simulink model "h2f_175_S2_sil_plant_model"  (R2023a)
settings: Solver=FixedStepAuto  StartTime=0.0  StopTime=10.0  FixedStep=0.02  RelTol=1e-3
PreLoadFcn:
  | addpath(fullfile('h175_model','thermal'))
  | run('thermal_variants_config.m')
undefined symbols (not defined in the file): b_AnodeSens, b_ARP1_SENS, b_ARP2_SENS, b_auxTCP_SENS, b_CathodeSens, b_CBV_SENS, b_CHUBVd_SENS, b_CHUBVw_SENS, b_CSIV_SENS, b_CSOV_SENS, b_EAC_SENS, b_EATBV_SENS, b_ECoolingSens, b_ElectricalSens, b_ETCP_SENS, b_ETV_SENS, b_ISens_BoP, b_mdotSens_EACi, b_pSens_APRVi, b_pSens_ASti, b_pSens_CLSti, b_pSens_ECL, b_RSens_ISOMON, b_Sens_IVT, b_StackRelay_SENS, b_TCP_SENS, b_TCV_SENS, b_ThermalSens, b_TSens_ASVi, b_TSens_CLSti, b_TSens_CLSto, b_TSens_CSti, b_TSens_TCVi, b_USens_StCV, clean_data_AnodeSens, clean_data_auxTCP_SENS, clean_data_CathodeSens, clean_data_EAC_SENS, clean_data_ECoolingSens, clean_data_ElectricalSens, clean_data_pSens_CLSti, clean_data_Sensors, clean_data_TCP_SENS, clean_data_TCV_SENS, clean_data_ThermalSens, clean_data_ThermalSim, clean_data_TSens_CLSti, clean_data_TSens_CLSto, clean_data_TSens_CSti, clean_data_TSens_TCVi, gaussian, init_Parameters, RELAY_STATE, s_I_A_BOP_Get, s_I_A_StN_Get, s_omega_rpm_ARP1_Get, s_omega_rpm_ARP2_Get, s_omega_rpm_EAC_Get, s_p_bara_APRVi_Get, s_p_bara_ASti_Get ... (+64)
libraries: simulink x17, nesl_utility x1
(part 1 of 2)
settings Model: Creator=stefan.notter  LastModifiedBy=stefan.notter
settings OptimizationCC: DefaultUnderspecifiedDataType=single  ReuseModelBlockBuffer=off
settings DebuggingCC: UnitsInconsistencyMsg=none

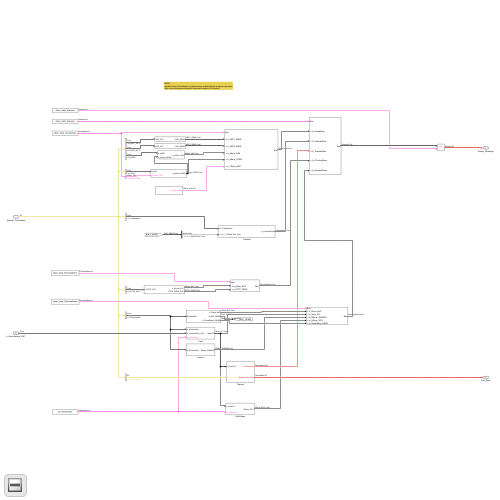
[thumbnail: Simulink's stored preview of the top-level diagram]
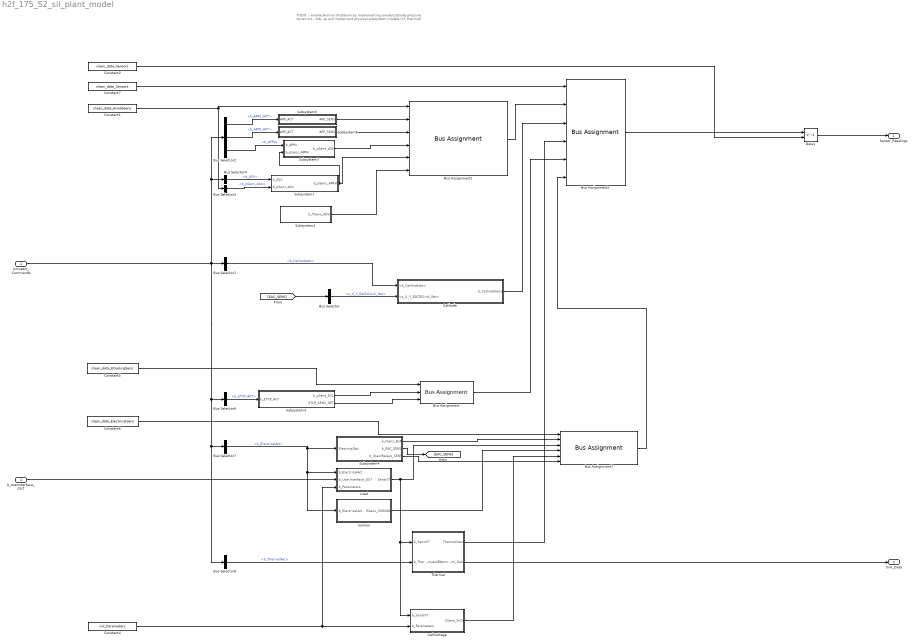
== system h2f_175_S2_sil_plant_model ==
  note: TODO:
      | - enable Normal Shutdown by implementing anode/cathode pressure dynamics
      | - tidy up and implement physical subsystem models (cf. thermal)
  Actuator_Commands : Inport  OutDataTypeStr=Bus: Actuators
  b_UserInterface_OUT : Inport  Port=2  OutDataTypeStr=Bus: UserInterface_OUT
  Bus Assignment : BusAssignment  AssignedSignals=b_pSens_ECL,b_ETCP_SENS
  Bus Assignment1 : BusAssignment  AssignedSignals=b_ARP1_SENS,b_ARP2_SENS,b_pSens_ASti,b_pSens_APRVi,b_TSens_ASVi
  Bus Assignment2 : BusAssignment  AssignedSignals=b_AnodeSens,b_CathodeSens,b_ThermalSens,b_ECoolingSens,b_ElectricalSens
  Bus Assignment7 : BusAssignment  AssignedSignals=b_ISens_BoP,b_Sens_IVT,b_RSens_ISOMON,b_USens_StCV,b_StackRelay_SENS
  Bus Selector : BusSelector  OutputSignals=s_U_V_EACDCLink_Get
  Bus Selector1 : BusSelector  OutputSignals=b_CathodeAct
  Bus Selector2 : BusSelector  OutputSignals=b_AnodeAct.b_ARP1_ACT,b_AnodeAct.b_ARP2_ACT,b_AnodeAct.b_APRV
  Bus Selector3 : BusSelector  OutputSignals=b_pSens_ASti
  Bus Selector4 : BusSelector  OutputSignals=b_AnodeAct.b_ASV
  Bus Selector6 : BusSelector  OutputSignals=b_ECoolingAct.b_ETCP_ACT
  Bus Selector7 : BusSelector  OutputSignals=b_ElectricalAct
  Bus Selector8 : BusSelector  OutputSignals=b_ThermalAct
  Cathode : Subsystem
  CellVoltage : Subsystem
  Constant1 : Constant  Value=clean_data_AnodeSens  OutDataTypeStr=Bus: AnodeSens
  Constant2 : Constant  Value=clean_data_Sensors  OutDataTypeStr=Bus: Sensors
  Constant4 : Constant  Value=init_Parameters  OutDataTypeStr=Bus: Parameters
  Constant5 : Constant  Value=clean_data_ECoolingSens  OutDataTypeStr=Bus: ECoolingSens
  Constant6 : Constant  Value=clean_data_ElectricalSens  OutDataTypeStr=Bus: ElectricalSens
  Constant7 : Constant  Value=clean_data_Sensors  OutDataTypeStr=Bus: Sensors
  Delay : Delay  DelayLength=1  InitialConditionSource=Input port
      settings: InputPortMap=u0,p4
  Isomon : Subsystem
  Load : Subsystem
  Subsystem1 : Subsystem
  Subsystem2 : Subsystem
  Subsystem3 : Subsystem
  Subsystem4 : Subsystem
  Subsystem5 : Subsystem
  Subsystem6 : Subsystem
  Subsystem7 : Subsystem
  Thermal : Subsystem
  Sensor_Readings : Outport  OutDataTypeStr=Bus: Sensors
  Sim_Data : Outport  Port=2  OutDataTypeStr=Bus: ThermalSim
  wires:
  Bus Selector2/2 -> Subsystem6/1(ARP_ACT)  "<b_ARP2_ACT>"
  Constant4/1 -> Load/3(b_Parameters), CellVoltage/2(b_Parameters)
  CellVoltage/1(USens_StCV) -> Bus Assignment7/5
  Isomon/1(RSens_ISOMON) -> Bus Assignment7/4
  Subsystem4/2(b_EAC_SENS) -> [EAC_SENS]
  Constant6/1 -> Bus Assignment7/1
  Subsystem3/2(ETCP_SENS_GET) -> Bus Assignment/3
  Delay/1 -> Sensor_Readings/1
  b_UserInterface_OUT/1 -> Load/2(b_UserInterface_OUT)
  Bus Selector4/1 -> Subsystem1/1(b_ASV)  "<b_ASV>"
  Constant1/1 -> Bus Selector3/1, Bus Assignment1/1
  Load/1(SensIVT) -> CellVoltage/1(b_SensIVT), Thermal/1(b_SensIVT), Bus Assignment7/3
  Bus Assignment2/1 -> Delay/1
  Subsystem3/1(b_pSens_ECL) -> Bus Assignment/2
  Bus Assignment1/1 -> Bus Assignment2/2
  Bus Assignment/1 -> Bus Assignment2/5
  Thermal/1(ThermalSens) -> Bus Assignment2/4
  Bus Selector2/1 -> Subsystem5/1(ARP_ACT)  "<b_ARP1_ACT>"
  Subsystem6/1(ARP_SENS) -> Bus Assignment1/3
  Constant2/1 -> Delay/2
  Subsystem5/1(ARP_SENS) -> Bus Assignment1/2
  Bus Selector8/1 -> Thermal/2(b_ThermalActuators)  "<b_ThermalAct>"
  Actuator_Commands/1 -> Bus Selector1/1, Bus Selector2/1, Bus Selector4/1, Bus Selector8/1, Bus Selector7/1, Bus Selector6/1
  Constant5/1 -> Bus Assignment/1
  Constant7/1 -> Bus Assignment2/1
  Bus Assignment7/1 -> Bus Assignment2/6
  Bus Selector3/1 -> Subsystem1/2(b_pSens_ASti)  "<b_pSens_ASti>"
  Bus Selector7/1 -> Subsystem4/1(ElectricalAct), Isomon/1(b_ElectricalAct), Load/1(b_ElectricalAct)  "<b_ElectricalAct>"
  Bus Selector6/1 -> Subsystem3/1(b_ETCP_ACT)  "<b_ETCP_ACT>"
  Subsystem1/1(b_pSens_APRVi) -> Subsystem7/2(b_pSens_APRVi), Bus Assignment1/5
  Subsystem4/1(b_ISens_BoP) -> Bus Assignment7/2
  [EAC_SENS] -> Bus Selector/1
  Subsystem4/3(b_StackRelays_SENS) -> Bus Assignment7/6
  Subsystem2/1(b_TSens_ASVi) -> Bus Assignment1/6
  Bus Selector2/3 -> Subsystem7/1(b_APRV)  "<b_APRV>"
  Subsystem7/1(b_pSens_ASti) -> Bus Assignment1/4
  Bus Selector1/1 -> Cathode/1(<b_CathodeAct>)  "<b_CathodeAct>"
  Bus Selector/1 -> Cathode/2(<s_U_V_EACDCLink_Get>)  "<s_U_V_EACDCLink_Get>"
  Cathode/1(b_CathodeSens) -> Bus Assignment2/3
  Thermal/2(Thermal_Sim_Data) -> Sim_Data/1

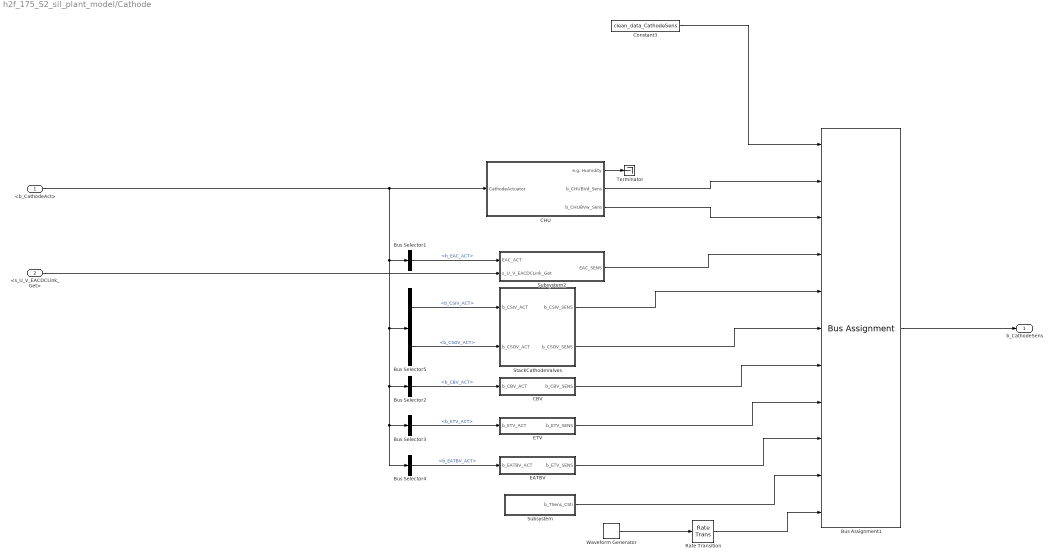
== system h2f_175_S2_sil_plant_model/Cathode ==
  <b_CathodeAct> : Inport
  <s_U_V_EACDCLink_Get> : Inport  Port=2
  Bus Assignment1 : BusAssignment  AssignedSignals=b_CHUBVd_SENS,b_CHUBVw_SENS,b_EAC_SENS,b_CSIV_SENS,b_CSOV_SENS,b_CBV_SENS,b_ETV_SENS,b_EATBV_SENS,b_TSens_CSti,b_mdotSens_EACi.s_mDot_gps_EACi_Get
  Bus Selector1 : BusSelector  OutputSignals=b_EAC_ACT
  Bus Selector2 : BusSelector  OutputSignals=b_CBV_ACT
  Bus Selector3 : BusSelector  OutputSignals=b_ETV_ACT
  Bus Selector4 : BusSelector  OutputSignals=b_EATBV_ACT
  Bus Selector5 : BusSelector  OutputSignals=b_CSIV_ACT,b_CSOV_ACT
  CBV : Subsystem
  CHU : Subsystem
  Constant3 : Constant  Value=clean_data_CathodeSens  OutDataTypeStr=Bus: CathodeSens
  EATBV : Subsystem
  ETV : Subsystem
  Rate Transition : RateTransition
  StackCathodeValves : Subsystem
  Subsystem : Subsystem
  Subsystem2 : Subsystem
  Terminator : Terminator
  Waveform Generator : simulink/Sources/Waveform Generator  OutMin=[]  OutMax=[]  OutDataTypeStr=single  SelectedSignal=1  Signals=gaussian(200,6,23)  BlockNames=MultiportSwitch_9f1233eeb05b44e  SampleTime=0.1
  b_CathodeSens : Outport
  wires:
  Bus Assignment1/1 -> b_CathodeSens/1
  Waveform Generator/1 -> Rate Transition/1
  EATBV/1(b_ETV_SENS) -> Bus Assignment1/9
  Bus Selector4/1 -> EATBV/1(b_EATBV_ACT)  "<b_EATBV_ACT>"
  ETV/1(b_ETV_SENS) -> Bus Assignment1/8
  Subsystem/1(b_TSens_CSti) -> Bus Assignment1/10
  CHU/2(b_CHUBVd_Sens) -> Bus Assignment1/2
  Rate Transition/1 -> Bus Assignment1/11
  StackCathodeValves/1(b_CSIV_SENS) -> Bus Assignment1/5
  StackCathodeValves/2(b_CSOV_SENS) -> Bus Assignment1/6
  Bus Selector2/1 -> CBV/1(b_CBV_ACT)  "<b_CBV_ACT>"
  Bus Selector5/1 -> StackCathodeValves/1(b_CSIV_ACT)  "<b_CSIV_ACT>"
  Bus Selector1/1 -> Subsystem2/1(EAC_ACT)  "<b_EAC_ACT>"
  Bus Selector5/2 -> StackCathodeValves/2(b_CSOV_ACT)  "<b_CSOV_ACT>"
  Bus Selector3/1 -> ETV/1(b_ETV_ACT)  "<b_ETV_ACT>"
  CHU/1(e.g. Humidity) -> Terminator/1
  Subsystem2/1(EAC_SENS) -> Bus Assignment1/4
  <s_U_V_EACDCLink_Get>/1 -> Subsystem2/2(s_U_V_EACDCLink_Get)
  Constant3/1 -> Bus Assignment1/1
  <b_CathodeAct>/1 -> CHU/1(CathodeActuator), Bus Selector1/1, Bus Selector5/1, Bus Selector2/1, Bus Selector3/1, Bus Selector4/1
  CHU/3(b_CHUBVw_Sens) -> Bus Assignment1/3
  CBV/1(b_CBV_SENS) -> Bus Assignment1/7

== system h2f_175_S2_sil_plant_model/CellVoltage ==
  b_SensIVT : Inport  OutDataTypeStr=Bus: Sens_IVT
  b_Parameters : Inport  Port=2  OutDataTypeStr=Bus: Parameters
  Bus Assignment : BusAssignment  AssignedSignals=s_U_V_CVAVG_Get,s_U_V_CVMAX_Get,s_U_V_CVMIN_Get,s_st_enum_StCV_Get
  Bus Selector : BusSelector  OutputSignals=s_U_V_StP_Get
  Bus Selector1 : BusSelector  OutputSignals=b_GEN_Parameters.p_NumberOfCells
  Constant : Constant  Value=struct_USens_StCV  OutDataTypeStr=Bus: USens_StCV
  Divide : Product  Inputs=*/
  Enumerated Constant : simulink/Sources/Enumerated Constant  OutDataTypeStr=Enum: SENS_STATUS  Value=SENS_STATUS.OK  SampleTime=inf
  Gain1 : Gain  Gain=1.01
  Gain2 : Gain  Gain=0.99
  USens_StCV : Outport  OutDataTypeStr=Bus: USens_StCV
  wires:
  Constant/1 -> Bus Assignment/1
  Bus Assignment/1 -> USens_StCV/1
  b_SensIVT/1 -> Bus Selector/1
  Bus Selector/1 -> Divide/1  "<s_U_V_StP_Get>"
  Gain1/1 -> Bus Assignment/3
  Gain2/1 -> Bus Assignment/4
  b_Parameters/1 -> Bus Selector1/1
  Bus Selector1/1 -> Divide/2  "<p_NumberOfCells>"
  Enumerated Constant/1 -> Bus Assignment/5
  Divide/1 -> Gain2/1, Gain1/1, Bus Assignment/2

== system h2f_175_S2_sil_plant_model/Isomon ==
  b_ElectricalAct : Inport  OutDataTypeStr=Bus: ElectricalAct
  Bus Assignment : BusAssignment  AssignedSignals=s_State_enum_ISOMON_Get,s_R_Ohm_ISOMON_Get
  Bus Selector : BusSelector  OutputSignals=b_RSens_ISOMON_ACT.s_State_enum_ISOMON_Set
  Constant : Constant  Value=struct_RSens_ISOMON  OutDataTypeStr=Bus: RSens_ISOMON
  Constant1 : Constant  Value=5e4  OutDataTypeStr=single
  RSens_ISOMON : Outport  OutDataTypeStr=Bus: RSens_ISOMON
  wires:
  Bus Selector/1 -> Bus Assignment/2  "<s_State_enum_ISOMON_Set>"
  b_ElectricalAct/1 -> Bus Selector/1
  Bus Assignment/1 -> RSens_ISOMON/1
  Constant/1 -> Bus Assignment/1
  Constant1/1 -> Bus Assignment/3

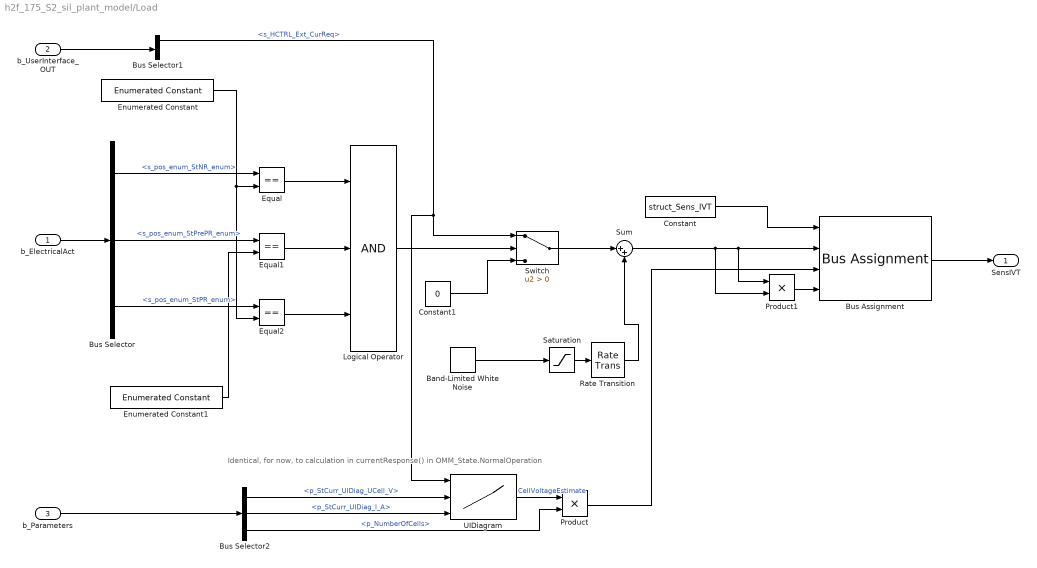
== system h2f_175_S2_sil_plant_model/Load ==
  note: Identical, for now, to calculation in currentResponse() in OMM_State.NormalOperation
  b_ElectricalAct : Inport  OutDataTypeStr=Bus: ElectricalAct
  b_UserInterface_OUT : Inport  Port=2  OutDataTypeStr=Bus: UserInterface_OUT
  b_Parameters : Inport  Port=3  OutDataTypeStr=Bus: Parameters
  Band-Limited White Noise : simulink/Sources/Band-Limited White Noise  Cov=[0.5]  Ts=0.1  seed=[23341]
  Bus Assignment : BusAssignment  AssignedSignals=s_I_A_StN_Get,s_U_V_StP_Get,s_P_W_St_Get
  Bus Selector : BusSelector  OutputSignals=b_StackRelays.s_pos_enum_StNR_enum,b_StackRelays.s_pos_enum_StPrePR_enum,b_StackRelays.s_pos_enum_StPR_enum
  Bus Selector1 : BusSelector  OutputSignals=s_HCTRL_Ext_CurReq,s_HCTRL_Ext_MaxPow
  Bus Selector2 : BusSelector  OutputSignals=b_GEN_Parameters.p_StCurr_UIDiag_UCell_V,b_GEN_Parameters.p_StCurr_UIDiag_I_A,b_GEN_Parameters.p_NumberOfCells
  Constant : Constant  Value=struct_Sens_IVT  OutDataTypeStr=Bus: Sens_IVT
  Constant1 : Constant  Value=0
  Enumerated Constant : simulink/Sources/Enumerated Constant  OutDataTypeStr=Enum: RELAY_STATE  Value=RELAY_STATE.Connected  SampleTime=inf
  Enumerated Constant1 : simulink/Sources/Enumerated Constant  OutDataTypeStr=Enum: RELAY_STATE  Value=RELAY_STATE.Disconnected  SampleTime=inf
  Equal : RelationalOperator  Operator===  OutDataTypeStr=boolean  RndMeth=Simplest  InputSameDT=off
  Equal1 : RelationalOperator  Operator===  OutDataTypeStr=boolean  RndMeth=Simplest  InputSameDT=off
  Equal2 : RelationalOperator  Operator===  OutDataTypeStr=boolean  RndMeth=Simplest  InputSameDT=off
  Logical Operator : Logic  Inputs=3  AllPortsSameDT=off  OutDataTypeStr=boolean
  Product : Product
  Product1 : Product
  Rate Transition : RateTransition
  Saturation : Saturate  UpperLimit=0.4  LowerLimit=-0.4
  Sum : Sum  Inputs=|++  OutDataTypeStr=single
  Switch : Switch  Criteria=u2 > Threshold  SaturateOnIntegerOverflow=off  InputSameDT=off
  UIDiagram : Lookup_n-D  NumberOfTableDimensions=1  BreakpointsForDimension1Source=Input port  BreakpointsForDimension1=[-5:5]  BreakpointsForDimension2Source=Input port  TableSource=Input port  Table=tanh([-5:5])  ExtrapMethod=Clip  UseLastTableValue=on  InternalRulePriority=Speed  RndMeth=Simplest
      settings: InputPortMap=u0,p221,p5
  SensIVT : Outport  OutDataTypeStr=Bus: Sens_IVT
  wires:
  Constant/1 -> Bus Assignment/1
  Bus Assignment/1 -> SensIVT/1
  b_ElectricalAct/1 -> Bus Selector/1
  Constant1/1 -> Switch/3
  Sum/1 -> Product1/2, Product1/1, Bus Assignment/2
  Bus Selector/2 -> Equal1/1  "<s_pos_enum_StPrePR_enum>"
  Bus Selector/3 -> Equal2/1  "<s_pos_enum_StPR_enum>"
  Bus Selector/1 -> Equal/1  "<s_pos_enum_StNR_enum>"
  Equal/1 -> Logical Operator/1
  Equal1/1 -> Logical Operator/2
  Equal2/1 -> Logical Operator/3
  Enumerated Constant/1 -> Equal2/2, Equal/2
  Enumerated Constant1/1 -> Equal1/2
  Logical Operator/1 -> Switch/2
  b_UserInterface_OUT/1 -> Bus Selector1/1
  Bus Selector1/1 -> UIDiagram/1, Switch/1  "<s_HCTRL_Ext_CurReq>"
  b_Parameters/1 -> Bus Selector2/1
  Bus Selector2/2 -> UIDiagram/3  "<p_StCurr_UIDiag_I_A>"
  Bus Selector2/1 -> UIDiagram/2  "<p_StCurr_UIDiag_UCell_V>"
  UIDiagram/1 -> Product/1  "CellVoltageEstimate"
  Bus Selector2/3 -> Product/2  "<p_NumberOfCells>"
  Product/1 -> Bus Assignment/3
  Product1/1 -> Bus Assignment/4
  Band-Limited White Noise/1 -> Saturation/1
  Switch/1 -> Sum/1
  Rate Transition/1 -> Sum/2
  Saturation/1 -> Rate Transition/1

== system h2f_175_S2_sil_plant_model/Subsystem1 ==
  b_ASV : Inport  OutDataTypeStr=Bus: ASV  PortDimensions=1
  b_pSens_ASti : Inport  Port=2  OutDataTypeStr=Bus: pSens_ASti  PortDimensions=1
  Bus Assignment : BusAssignment  AssignedSignals=s_p_bara_APRVi_Get,s_st_enum_APRVi_Get
  Bus Selector : BusSelector  OutputSignals=s_pos_enum_ASV_Set
  Bus Selector1 : BusSelector  OutputSignals=s_p_bara_ASti_Get
  Constant : Constant  Value=struct_pSens_APRVi  OutDataTypeStr=Bus: pSens_APRVi
  Enumerated Constant : simulink/Sources/Enumerated Constant  OutDataTypeStr=Enum: SENS_STATUS  Value=SENS_STATUS.OK  SampleTime=inf
  Multiport Switch : MultiPortSwitch  DataPortOrder=Specify indices  DataPortIndices={DVLV_STATE.Open, DVLV_STATE.Closed}  SaturateOnIntegerOverflow=off  InputSameDT=off
  Sum : Sum  Inputs=|++
  bara : Constant  Value=2.79  OutDataTypeStr=single
  dontJudge : Constant  Value=3  OutDataTypeStr=single
  b_pSens_APRVi : Outport  OutDataTypeStr=Bus: pSens_APRVi
  wires:
  Constant/1 -> Bus Assignment/1
  bara/1 -> Multiport Switch/2
  Enumerated Constant/1 -> Bus Assignment/3
  Bus Selector/1 -> Multiport Switch/1  "<s_pos_enum_ASV_Set>"
  Bus Assignment/1 -> b_pSens_APRVi/1
  Multiport Switch/1 -> Bus Assignment/2
  b_pSens_ASti/1 -> Bus Selector1/1
  Sum/1 -> Multiport Switch/3
  b_ASV/1 -> Bus Selector/1
  Bus Selector1/1 -> Sum/1  "<s_p_bara_ASti_Get>"
  dontJudge/1 -> Sum/2

== system h2f_175_S2_sil_plant_model/Subsystem2 ==
  Bus Assignment : BusAssignment  AssignedSignals=s_T_degC_ASVi_Get,s_st_enum_ASVi_Get
  Constant : Constant  Value=30  OutDataTypeStr=single
  Constant1 : Constant  Value=struct_TSens_ASVi  OutDataTypeStr=Bus: TSens_ASVi
  Enumerated Constant : simulink/Sources/Enumerated Constant  OutDataTypeStr=Enum: SENS_STATUS  Value=SENS_STATUS.OK  SampleTime=inf
  b_TSens_ASVi : Outport
  wires:
  Constant/1 -> Bus Assignment/2
  Enumerated Constant/1 -> Bus Assignment/3
  Constant1/1 -> Bus Assignment/1
  Bus Assignment/1 -> b_TSens_ASVi/1

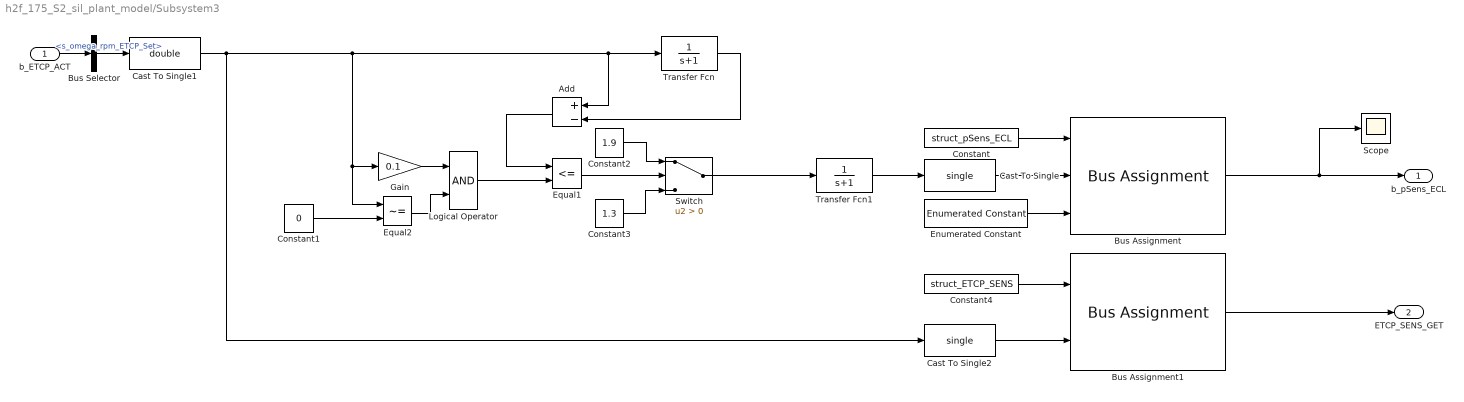
== system h2f_175_S2_sil_plant_model/Subsystem3 ==
  b_ETCP_ACT : Inport  OutDataTypeStr=Bus: ETCP_ACT
  Add : Sum  Inputs=+-
  Bus Assignment : BusAssignment  AssignedSignals=s_p_bara_ECL_Get,s_st_enum_ECL_Get
  Bus Assignment1 : BusAssignment  AssignedSignals=s_omega_rpm_ETCP_Get
  Bus Selector : BusSelector  OutputSignals=s_omega_rpm_ETCP_Set
  Cast To Single : DataTypeConversion  OutDataTypeStr=single  SaturateOnIntegerOverflow=off  RndMeth=Floor
  Cast To Single1 : DataTypeConversion  OutDataTypeStr=double  SaturateOnIntegerOverflow=off  RndMeth=Floor
  Cast To Single2 : DataTypeConversion  OutDataTypeStr=single  SaturateOnIntegerOverflow=off  RndMeth=Floor
  Constant : Constant  Value=struct_pSens_ECL  OutDataTypeStr=Bus: pSens_ECL
  Constant1 : Constant  Value=0
  Constant2 : Constant  Value=1.9
  Constant3 : Constant  Value=1.3
  Constant4 : Constant  Value=struct_ETCP_SENS  OutDataTypeStr=Bus: ETCP_SENS
  Enumerated Constant : simulink/Sources/Enumerated Constant  OutDataTypeStr=Enum: SENS_STATUS  Value=SENS_STATUS.OK  SampleTime=inf
  Equal1 : RelationalOperator  Operator=<=  OutDataTypeStr=boolean  RndMeth=Simplest  InputSameDT=off
  Equal2 : RelationalOperator  Operator=~=  OutDataTypeStr=boolean  RndMeth=Simplest  InputSameDT=off
  Gain : Gain  Gain=0.1
  Logical Operator : Logic  AllPortsSameDT=off  OutDataTypeStr=boolean
  Scope : Scope
  Switch : Switch  Criteria=u2 > Threshold  SaturateOnIntegerOverflow=off  InputSameDT=off
  Transfer Fcn : TransferFcn  Denominator=[1 1]
  Transfer Fcn1 : TransferFcn  Denominator=[1 1]
  b_pSens_ECL : Outport  OutDataTypeStr=Bus: pSens_ECL
  ETCP_SENS_GET : Outport  Port=2  OutDataTypeStr=Bus: ETCP_SENS
  wires:
  Bus Selector/1 -> Cast To Single1/1  "<s_omega_rpm_ETCP_Set>"
  Constant1/1 -> Equal2/2
  Switch/1 -> Transfer Fcn1/1
  b_ETCP_ACT/1 -> Bus Selector/1
  Constant2/1 -> Switch/1
  Logical Operator/1 -> Equal1/2
  Transfer Fcn1/1 -> Cast To Single/1
  Equal2/1 -> Logical Operator/2
  Equal1/1 -> Switch/2
  Constant3/1 -> Switch/3
  Gain/1 -> Logical Operator/1
  Add/1 -> Equal1/1
  Constant4/1 -> Bus Assignment1/1
  Bus Assignment/1 -> Scope/1, b_pSens_ECL/1
  Enumerated Constant/1 -> Bus Assignment/3
  Bus Assignment1/1 -> ETCP_SENS_GET/1
  Constant/1 -> Bus Assignment/1
  Transfer Fcn/1 -> Add/2
  Cast To Single/1 -> Bus Assignment/2
  Cast To Single1/1 -> Cast To Single2/1, Equal2/1, Gain/1, Add/1, Transfer Fcn/1
  Cast To Single2/1 -> Bus Assignment1/2

== system h2f_175_S2_sil_plant_model/Subsystem4 ==
  ElectricalAct : Inport  OutDataTypeStr=Bus: ElectricalAct
  HVRelays : Subsystem
  StackRelays : Subsystem
  b_ISens_BoP : Outport  OutDataTypeStr=Bus: ISens_BoP
  b_EAC_SENS : Outport  Port=2  OutDataTypeStr=Bus: EAC_SENS
  b_StackRelays_SENS : Outport  Port=3  OutDataTypeStr=Bus: StackRelay_SENS
  wires:
  ElectricalAct/1 -> HVRelays/1(ElectricalAct), StackRelays/1(ElectricalAct)
  StackRelays/1(b_ISens_BoP) -> b_ISens_BoP/1
  HVRelays/1(b_EAC_SENS) -> b_EAC_SENS/1
  StackRelays/2(b_StackRelays_SENS) -> b_StackRelays_SENS/1

== system h2f_175_S2_sil_plant_model/Subsystem5 ==
  ARP_ACT : Inport  OutDataTypeStr=Bus: ARP1_ACT  PortDimensions=1
  Bus Assignment : BusAssignment  AssignedSignals=s_omega_rpm_ARP1_Get,s_st_enum_ARP1_Get
  Bus Selector : BusSelector  OutputSignals=s_omega_rpm_ARP1_Set
  Cast To Double : DataTypeConversion  OutDataTypeStr=double  SaturateOnIntegerOverflow=off  RndMeth=Floor
  Cast To Single : DataTypeConversion  OutDataTypeStr=single  SaturateOnIntegerOverflow=off  RndMeth=Floor
  Constant : Constant  Value=struct_ARP1_SENS  OutDataTypeStr=Bus: ARP1_SENS
  Enumerated Constant : simulink/Sources/Enumerated Constant  OutDataTypeStr=Enum: SENS_STATUS  Value=SENS_STATUS.OK  SampleTime=inf
  Transfer Fcn : TransferFcn  Numerator=[4]  Denominator=[1 2 4]
  ARP_SENS : Outport  OutDataTypeStr=Bus: ARP1_SENS  PortDimensions=1
  wires:
  Bus Assignment/1 -> ARP_SENS/1
  Enumerated Constant/1 -> Bus Assignment/3
  Bus Selector/1 -> Cast To Double/1  "<s_omega_rpm_ARP1_Set>"
  ARP_ACT/1 -> Bus Selector/1
  Constant/1 -> Bus Assignment/1
  Transfer Fcn/1 -> Cast To Single/1  "meas"
  Cast To Single/1 -> Bus Assignment/2
  Cast To Double/1 -> Transfer Fcn/1

== system h2f_175_S2_sil_plant_model/Subsystem6 ==
  ARP_ACT : Inport  OutDataTypeStr=Bus: ARP2_ACT  PortDimensions=1
  Bus Assignment : BusAssignment  AssignedSignals=s_omega_rpm_ARP2_Get,s_st_enum_ARP2_Get
  Bus Selector : BusSelector  OutputSignals=s_omega_rpm_ARP2_Set
  Cast To Double : DataTypeConversion  OutDataTypeStr=double  SaturateOnIntegerOverflow=off  RndMeth=Floor
  Cast To Single : DataTypeConversion  OutDataTypeStr=single  SaturateOnIntegerOverflow=off  RndMeth=Floor
  Constant : Constant  Value=struct_ARP2_SENS  OutDataTypeStr=Bus: ARP2_SENS
  Enumerated Constant : simulink/Sources/Enumerated Constant  OutDataTypeStr=Enum: SENS_STATUS  Value=SENS_STATUS.OK  SampleTime=inf
  Transfer Fcn : TransferFcn  Numerator=[4]  Denominator=[1 2 4]
  ARP_SENS : Outport  OutDataTypeStr=Bus: ARP2_SENS  PortDimensions=1
  wires:
  Transfer Fcn/1 -> Cast To Single/1  "meas"
  Enumerated Constant/1 -> Bus Assignment/3
  ARP_ACT/1 -> Bus Selector/1
  Constant/1 -> Bus Assignment/1
  Bus Selector/1 -> Cast To Double/1  "<s_omega_rpm_ARP2_Set>"
  Bus Assignment/1 -> ARP_SENS/1
  Cast To Double/1 -> Transfer Fcn/1
  Cast To Single/1 -> Bus Assignment/2

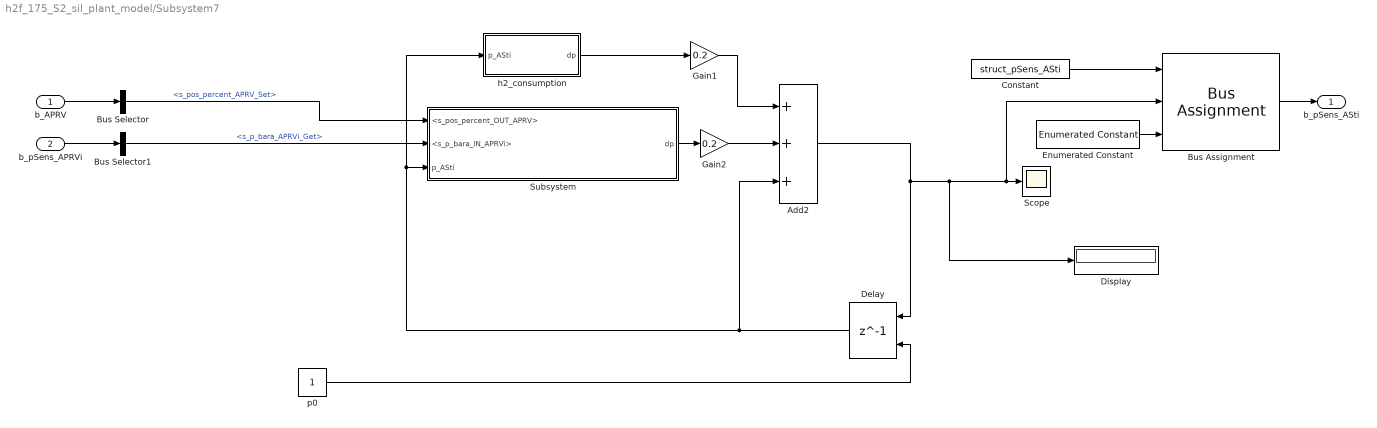
== system h2f_175_S2_sil_plant_model/Subsystem7 ==
  b_APRV : Inport  OutDataTypeStr=Bus: APRV  PortDimensions=1
  b_pSens_APRVi : Inport  Port=2  OutDataTypeStr=Bus: pSens_APRVi  PortDimensions=1
  Add2 : Sum  Inputs=+++
  Bus Assignment : BusAssignment  AssignedSignals=s_p_bara_ASti_Get,s_st_enum_ASti_Get
  Bus Selector : BusSelector  OutputSignals=s_pos_percent_APRV_Set
  Bus Selector1 : BusSelector  OutputSignals=s_p_bara_APRVi_Get
  Constant : Constant  Value=struct_pSens_ASti  OutDataTypeStr=Bus: pSens_ASti
  Delay : Delay  DelayLength=1  InitialConditionSource=Input port
      settings: InputPortMap=u0,p4
  Display : Display
  Enumerated Constant : simulink/Sources/Enumerated Constant  OutDataTypeStr=Enum: SENS_STATUS  Value=SENS_STATUS.OK  SampleTime=inf
  Gain1 : Gain  Gain=0.2
  Gain2 : Gain  Gain=0.2
  Scope : Scope
  Subsystem : Subsystem
  h2_consumption : Subsystem
  p0 : Constant  OutDataTypeStr=single
  b_pSens_ASti : Outport  OutDataTypeStr=Bus: pSens_ASti
  wires:
  Enumerated Constant/1 -> Bus Assignment/3
  h2_consumption/1(dp) -> Gain1/1
  Subsystem/1(dp) -> Gain2/1
  Constant/1 -> Bus Assignment/1
  Bus Selector/1 -> Subsystem/1(<s_pos_percent_OUT_APRV>)  "<s_pos_percent_APRV_Set>"
  Bus Selector1/1 -> Subsystem/2(<s_p_bara_IN_APRVi>)  "<s_p_bara_APRVi_Get>"
  Delay/1 -> h2_consumption/1(p_ASti), Subsystem/3(p_ASti), Add2/3
  p0/1 -> Delay/2
  b_pSens_APRVi/1 -> Bus Selector1/1
  Bus Assignment/1 -> b_pSens_ASti/1
  b_APRV/1 -> Bus Selector/1
  Add2/1 -> Delay/1, Display/1, Scope/1, Bus Assignment/2
  Gain1/1 -> Add2/1
  Gain2/1 -> Add2/2

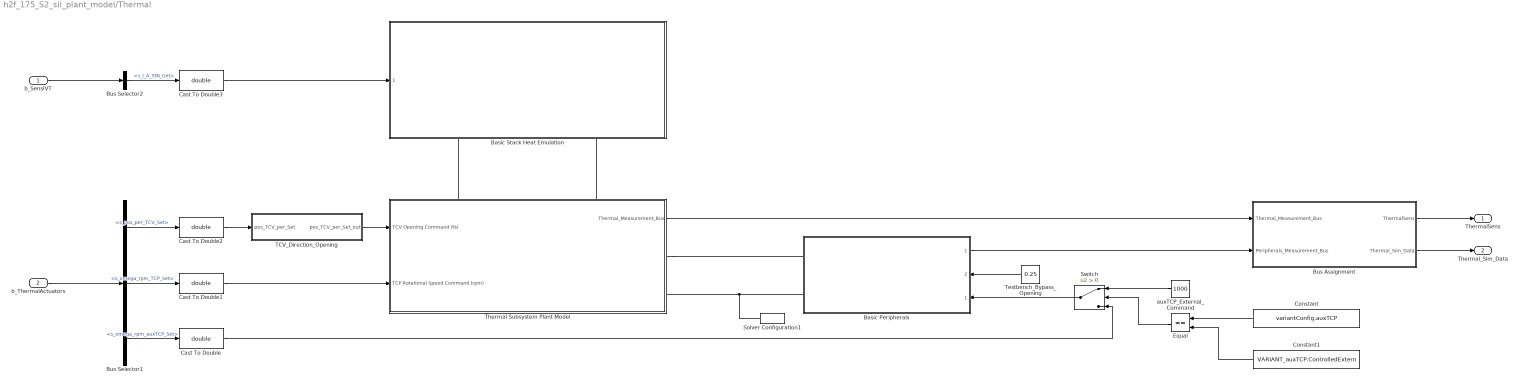
== system h2f_175_S2_sil_plant_model/Thermal ==
  b_SensIVT : Inport
  b_ThermalActuators : Inport  Port=2  OutDataTypeStr=Bus: ThermalAct
  Basic Peripherals : Subsystem  ReferencedSubsystem=thermal_basic_peripherals
      settings: PortSchema="{\"entries\":[{\"content\":{\"sides\":[{\"content\":{\"connectorIds\":[\"LConn1\",\"LConn2\"]},\"type\":\"ConnectorPlacement.EquallySpacedRectSide\",\"uuid\":\"3fb1bffc-06de-43a0-ba54-014616fc6cc1\"},{\"content\":{\"connectorIds\":[\"Out1\",\"In2\",\"In1\"],\"side\":\"RIGHT\"},\"type\":\"ConnectorPlacement.EquallySpacedRectSide\",\"uuid\":\"58405954-0a26-4c47-92cd-2c539f5c2dc2\"},{\"content\":{\"side\":\"TOP\"},\"type\":\"ConnectorPlacement.EquallySpacedRectSide\",\"uuid\":\"fb935e14-bdb8-42f8-ab88-5e819e25323e\"},{\"content\":{\"side\":\"BOTTOM\"},\"type\":\"ConnectorPlacement.EquallySpacedRectSide\",\"uuid\":\"e6e8be2d-a7ad-4d02-9de8-873dcaf650b4\"}]},\"type\":\"ConnectorPlacement.EquallySpacedConnector\",\"uuid\":\"bd863423-caf1-4028-a014-0e522635d1ca\"}],\"packageUris\":[\"http://schema.mathworks.com/mf0/Connector/R2020b\"],\"version\":\"1.0\"}"
  Basic Stack Heat Emulation : Subsystem  ReferencedSubsystem=thermal_stack_heat_emulation
      settings: PortSchema="{\"entries\":[{\"content\":{\"sides\":[{\"content\":{\"connectorIds\":[\"In1\"]},\"type\":\"ConnectorPlacement.EquallySpacedRectSide\",\"uuid\":\"3fb1bffc-06de-43a0-ba54-014616fc6cc1\"},{\"content\":{\"side\":\"RIGHT\"},\"type\":\"ConnectorPlacement.EquallySpacedRectSide\",\"uuid\":\"58405954-0a26-4c47-92cd-2c539f5c2dc2\"},{\"content\":{\"side\":\"TOP\"},\"type\":\"ConnectorPlacement.EquallySpacedRectSide\",\"uuid\":\"fb935e14-bdb8-42f8-ab88-5e819e25323e\"},{\"content\":{\"connectorIds\":[\"RConn1\",\"RConn2\"],\"side\":\"BOTTOM\"},\"type\":\"ConnectorPlacement.EquallySpacedRectSide\",\"uuid\":\"52bc4db1-df79-4132-9e52-2843fbef2d40\"}]},\"type\":\"ConnectorPlacement.EquallySpacedConnector\",\"uuid\":\"bd863423-caf1-4028-a014-0e522635d1ca\"}],\"packageUris\":[\"http://schema.mathworks.com/mf0/Connector/R2020b\"],\"version\":\"1.0\"}"
  Bus Selector1 : BusSelector  OutputSignals=b_TCV_ACT.s_pos_per_TCV_Set,b_TCP_ACT.s_omega_rpm_TCP_Set,b_auxTCP_ACT.s_omega_rpm_auxTCP_Set
  Bus Selector2 : BusSelector  OutputSignals=s_I_A_StN_Get
  Bus Assignment : Subsystem
  Cast To Double{,1..3} (4 alike) : DataTypeConversion  OutDataTypeStr=double  SaturateOnIntegerOverflow=off  RndMeth=Floor
  Constant : Constant  Value=variantConfig.auxTCP
  Constant1 : Constant  Value=VARIANT_auxTCP.ControlledExtern
  Equal : RelationalOperator  Operator===  OutDataTypeStr=boolean  RndMeth=Simplest  InputSameDT=off
  Solver Configuration1 : nesl_utility/Solver Configuration  PhysicalDomain=network_engine_domain  SubClassName=solver  LeftPortType=input  RightPortType=generic  Tones=[]  Harmonics=[]  SimulateNoise=off  Profile=off  UseLocalSampling=off  EnableSwitchedLinearOptims=on  FrequencyDomain=off  UseCCode=off  RelTol=0.001  AbsTol=1e-06  MinStep=1e-09  ToWorkspace=off  RevertToSquareIcSolve=off  NumHomotopyIterations=100  PhasorMode=off  PhasorModeNumHarmonics=1  ConsistencySolver=NEWTON_XTOL_AFTER_FTOL  IndexReductionMethod=DerivativeReplacement  DoDC=off  ResidualTolerance=1e-09  ConsistencyTolSource=GLOBAL  ConsistencyAbsTol=0.001  ConsistencyRelTol=0.001  ConsistencyTolFactor=0.001  UseLocalSolver=on  LocalSolverChoice=NE_BACKWARD_EULER_ADVANCER  ResolveIndetEquations=on  FunctionEvalNumThread=1  LocalSolverSampleTime=0.02  DoFixedCost=on  MaxNonlinIter=3  MaxModeIter=2  ComputeImpulses=off  ImpulseIterations=2  LinearAlgebra=auto  LinearAlgebraNumThread=0  EquationFormulation=NE_TIME_EF  DelaysMemoryBudget=1024  AutomaticFiltering=off  FilteringTimeConstant=0.001  PartitionStorageMethod=AS_NEEDED  PartitionMemoryBudget=1024  PartitionMethod=ROBUST
  Switch : Switch  Criteria=u2 > Threshold  SaturateOnIntegerOverflow=off  InputSameDT=off
  TCV_Direction_Opening : Subsystem  Variant=on  VariantActivationTime=startup
  Testbench_Bypass_Opening : Constant  Value=0.25
  Thermal Subsystem Plant Model : Subsystem  Variant=on
      settings: PortSchema="{\"entries\":[{\"content\":{\"sides\":[{\"content\":{\"connectorIds\":[\"In1\",\"In2\"]},\"type\":\"ConnectorPlacement.EquallySpacedRectSide\",\"uuid\":\"c406812b-8c92-4602-a172-62ad771a81a9\"},{\"content\":{\"connectorIds\":[\"Out1\",\"RConn1\",\"RConn2\"],\"side\":\"RIGHT\"},\"type\":\"ConnectorPlacement.EquallySpacedRectSide\",\"uuid\":\"78b6fff5-4256-4005-adaa-354cc2ed5b7d\"},{\"content\":{\"connectorIds\":[\"LConn1\",\"LConn2\"],\"side\":\"TOP\"},\"type\":\"ConnectorPlacement.EquallySpacedRectSide\",\"uuid\":\"1d5f4f72-4393-4f38-b9ce-f5bde53d6a3a\"}]},\"type\":\"ConnectorPlacement.EquallySpacedConnector\",\"uuid\":\"f62a8404-8485-4e42-883e-e8d18b630e2d\"}],\"packageUris\":[\"http://schema.mathworks.com/mf0/Connector/R2020b\"],\"version\":\"1.0\"}"
  auxTCP_External_Command : Constant  Value=1000
  ThermalSens : Outport  OutDataTypeStr=Bus: ThermalSens
  Thermal_Sim_Data : Outport  Port=2  OutDataTypeStr=Bus: ThermalSim
  wires:
  b_ThermalActuators/1 -> Bus Selector1/1
  b_SensIVT/1 -> Bus Selector2/1
  Bus Selector1/2 -> Cast To Double1/1  "<s_omega_rpm_TCP_Set>"
  Bus Selector1/1 -> Cast To Double2/1  "<s_pos_per_TCV_Set>"
  Bus Selector2/1 -> Cast To Double3/1  "<s_I_A_StN_Get>"
  Testbench_Bypass_Opening/1 -> Basic Peripherals/2
  Bus Selector1/3 -> Cast To Double/1  "<s_omega_rpm_auxTCP_Set>"
  Thermal Subsystem Plant Model/1(Thermal_Measurement_Bus) -> Bus Assignment/1(Thermal_Measurement_Bus)
  Bus Assignment/1(ThermalSens) -> ThermalSens/1
  Cast To Double1/1 -> Thermal Subsystem Plant Model/2(TCP Rotational Speed Command (rpm))
  Cast To Double3/1 -> Basic Stack Heat Emulation/1
  Basic Peripherals/1 -> Bus Assignment/2(Peripherals_Measurement_Bus)
  Constant/1 -> Equal/1
  Constant1/1 -> Equal/2
  Equal/1 -> Switch/2
  Cast To Double/1 -> Switch/3
  Switch/1 -> Basic Peripherals/1
  auxTCP_External_Command/1 -> Switch/1
  Cast To Double2/1 -> TCV_Direction_Opening/1(pos_TCV_per_Set)
  TCV_Direction_Opening/1(pos_TCV_per_Set_out) -> Thermal Subsystem Plant Model/1(TCV Opening Command (%))
  Bus Assignment/2(Thermal_Sim_Data) -> Thermal_Sim_Data/1
  connections:
  Thermal Subsystem Plant Model/LConn1 -- Basic Stack Heat Emulation/RConn1
  Thermal Subsystem Plant Model/LConn2 -- Basic Stack Heat Emulation/RConn2
  Thermal Subsystem Plant Model/RConn1 -- Basic Peripherals/LConn1
  Basic Peripherals/LConn2 -- Thermal Subsystem Plant Model/RConn2 -- Solver Configuration1/RConn1

== system h2f_175_S2_sil_plant_model/Cathode/CBV ==
  b_CBV_ACT : Inport  OutDataTypeStr=Bus: CBV_ACT
  Bus Assignment : BusAssignment  AssignedSignals=s_pos_percent_CBV_Get,s_st_enum_CBV_Get
  Bus Selector : BusSelector  OutputSignals=s_pos_percent_CBV_Set
  CBV : Subsystem  ReferencedSubsystem=OES_Valve
  Constant : Constant  Value=struct_CBV_SENS  OutDataTypeStr=Bus: CBV_SENS
  b_CBV_SENS : Outport  OutDataTypeStr=Bus: CBV_SENS
  wires:
  Bus Assignment/1 -> b_CBV_SENS/1
  Constant/1 -> Bus Assignment/1
  Bus Selector/1 -> CBV/1  "<s_pos_percent_CBV_Set>"
  b_CBV_ACT/1 -> Bus Selector/1
  CBV/2 -> Bus Assignment/3
  CBV/1 -> Bus Assignment/2

== system h2f_175_S2_sil_plant_model/Cathode/CHU ==
  CathodeActuator : Inport
  CHUBVdw_Dynamics : Subsystem
  HumidifierDynamics : Subsystem
  e.g. Humidity : Outport
  b_CHUBVd_Sens : Outport  Port=2  OutDataTypeStr=Bus: CHUBVd_SENS
  b_CHUBVw_Sens : Outport  Port=3  OutDataTypeStr=Bus: CHUBVw_SENS
  wires:
  HumidifierDynamics/1(e.g. Humidity) -> e.g. Humidity/1
  CHUBVdw_Dynamics/2(b_CHUBVw_Sens) -> b_CHUBVw_Sens/1
  CathodeActuator/1 -> CHUBVdw_Dynamics/1(CathodeActuator)
  CHUBVdw_Dynamics/1(b_CHUBVd_Sens) -> b_CHUBVd_Sens/1
  CHUBVdw_Dynamics/3(s_pos_percent_CHUBVd_Get) -> HumidifierDynamics/1(s_pos_percent_CHUBVd_Get)
  CHUBVdw_Dynamics/4(s_pos_percent_CHUBVw_Get) -> HumidifierDynamics/2(s_pos_percent_CHUBVw_Get)

== system h2f_175_S2_sil_plant_model/Cathode/EATBV ==
  b_EATBV_ACT : Inport  OutDataTypeStr=Bus: EATBV_ACT
  Bus Assignment : BusAssignment  AssignedSignals=s_pos_percent_EATBV_Get,s_st_enum_EATBV_Get
  Bus Selector : BusSelector  OutputSignals=s_pos_percent_EATBV_Set
  CBV : Subsystem  ReferencedSubsystem=OES_Valve
  Constant : Constant  Value=struct_EATBV_SENS  OutDataTypeStr=Bus: EATBV_SENS
  b_ETV_SENS : Outport  OutDataTypeStr=Bus: EATBV_SENS
  wires:
  Bus Assignment/1 -> b_ETV_SENS/1
  Constant/1 -> Bus Assignment/1
  Bus Selector/1 -> CBV/1  "<s_pos_percent_EATBV_Set>"
  b_EATBV_ACT/1 -> Bus Selector/1
  CBV/2 -> Bus Assignment/3
  CBV/1 -> Bus Assignment/2

== system h2f_175_S2_sil_plant_model/Cathode/ETV ==
  b_ETV_ACT : Inport  OutDataTypeStr=Bus: ETV_ACT
  Bus Assignment : BusAssignment  AssignedSignals=s_pos_percent_ETV_Get,s_st_enum_ETV_Get
  Bus Selector : BusSelector  OutputSignals=s_pos_percent_ETV_Set
  CBV : Subsystem  ReferencedSubsystem=OES_Valve
  Constant : Constant  Value=struct_ETV_SENS  OutDataTypeStr=Bus: ETV_SENS
  b_ETV_SENS : Outport  OutDataTypeStr=Bus: ETV_SENS
  wires:
  CBV/1 -> Bus Assignment/2
  CBV/2 -> Bus Assignment/3
  b_ETV_ACT/1 -> Bus Selector/1
  Bus Selector/1 -> CBV/1  "<s_pos_percent_ETV_Set>"
  Constant/1 -> Bus Assignment/1
  Bus Assignment/1 -> b_ETV_SENS/1

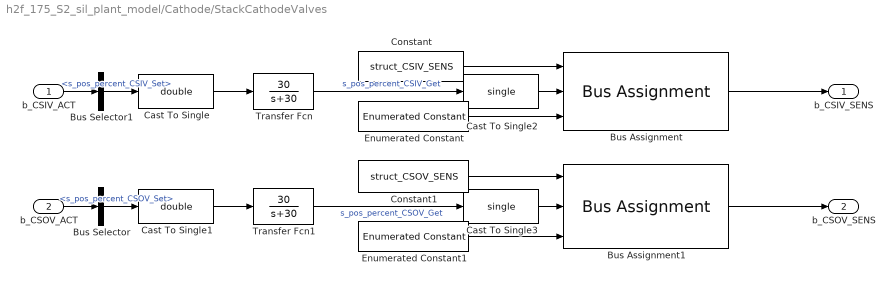
== system h2f_175_S2_sil_plant_model/Cathode/StackCathodeValves ==
  b_CSIV_ACT : Inport  OutDataTypeStr=Bus: CSIV_ACT
  b_CSOV_ACT : Inport  Port=2  OutDataTypeStr=Bus: CSOV_ACT
  Bus Assignment : BusAssignment  AssignedSignals=s_pos_percent_CSIV_Get,s_st_enum_CSIV_Get
  Bus Assignment1 : BusAssignment  AssignedSignals=s_pos_percent_CSOV_Get,s_st_enum_CSOV_Get
  Bus Selector : BusSelector  OutputSignals=s_pos_percent_CSOV_Set
  Bus Selector1 : BusSelector  OutputSignals=s_pos_percent_CSIV_Set
  Cast To Single : DataTypeConversion  OutDataTypeStr=double  SaturateOnIntegerOverflow=off  RndMeth=Floor
  Cast To Single1 : DataTypeConversion  OutDataTypeStr=double  SaturateOnIntegerOverflow=off  RndMeth=Floor
  Cast To Single2 : DataTypeConversion  OutDataTypeStr=single  SaturateOnIntegerOverflow=off  RndMeth=Floor
  Cast To Single3 : DataTypeConversion  OutDataTypeStr=single  SaturateOnIntegerOverflow=off  RndMeth=Floor
  Constant : Constant  Value=struct_CSIV_SENS  OutDataTypeStr=Bus: CSIV_SENS
  Constant1 : Constant  Value=struct_CSOV_SENS  OutDataTypeStr=Bus: CSOV_SENS
  Enumerated Constant : simulink/Sources/Enumerated Constant  OutDataTypeStr=Enum: SENS_STATUS  Value=SENS_STATUS.OK  SampleTime=inf
  Enumerated Constant1 : simulink/Sources/Enumerated Constant  OutDataTypeStr=Enum: SENS_STATUS  Value=SENS_STATUS.OK  SampleTime=inf
  Transfer Fcn : TransferFcn  Numerator=[30]  Denominator=[1 30]
  Transfer Fcn1 : TransferFcn  Numerator=[30]  Denominator=[1 30]
  b_CSIV_SENS : Outport
  b_CSOV_SENS : Outport  Port=2
  wires:
  Cast To Single3/1 -> Bus Assignment1/2
  Cast To Single2/1 -> Bus Assignment/2
  Cast To Single1/1 -> Transfer Fcn1/1
  Cast To Single/1 -> Transfer Fcn/1
  Enumerated Constant1/1 -> Bus Assignment1/3
  Enumerated Constant/1 -> Bus Assignment/3
  Bus Selector1/1 -> Cast To Single/1  "<s_pos_percent_CSIV_Set>"
  b_CSIV_ACT/1 -> Bus Selector1/1
  Bus Selector/1 -> Cast To Single1/1  "<s_pos_percent_CSOV_Set>"
  b_CSOV_ACT/1 -> Bus Selector/1
  Transfer Fcn1/1 -> Cast To Single3/1  "s_pos_percent_CSOV_Get"
  Transfer Fcn/1 -> Cast To Single2/1  "s_pos_percent_CSIV_Get"
  Bus Assignment1/1 -> b_CSOV_SENS/1
  Constant1/1 -> Bus Assignment1/1
  Bus Assignment/1 -> b_CSIV_SENS/1
  Constant/1 -> Bus Assignment/1

== system h2f_175_S2_sil_plant_model/Cathode/Subsystem ==
  Constant : Constant  Value=clean_data_TSens_CSti  OutDataTypeStr=Bus: TSens_CSti
  b_TSens_CSti : Outport  OutDataTypeStr=Bus: TSens_CSti
  wires:
  Constant/1 -> b_TSens_CSti/1

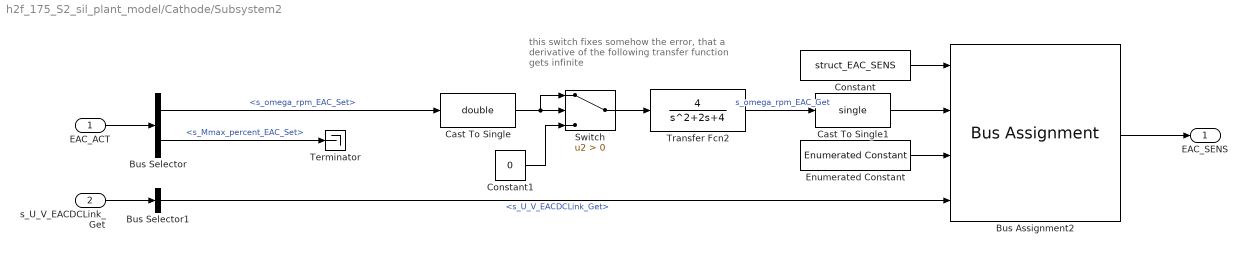
== system h2f_175_S2_sil_plant_model/Cathode/Subsystem2 ==
  note: this switch fixes somehow the error, that a derivative of the following transfer function gets infinite
  EAC_ACT : Inport  OutDataTypeStr=Bus: EAC_ACT  PortDimensions=1
  s_U_V_EACDCLink_Get : Inport  Port=2  OutDataTypeStr=single
  Bus Assignment2 : BusAssignment  AssignedSignals=s_omega_rpm_EAC_Get,s_st_enum_EAC_Get,s_U_V_EACDCLink_Get
  Bus Selector : BusSelector  OutputSignals=s_omega_rpm_EAC_Set,s_Mmax_percent_EAC_Set
  Bus Selector1 : BusSelector  OutputSignals=s_U_V_EACDCLink_Get
  Cast To Single : DataTypeConversion  OutDataTypeStr=double  SaturateOnIntegerOverflow=off  RndMeth=Floor
  Cast To Single1 : DataTypeConversion  OutDataTypeStr=single  SaturateOnIntegerOverflow=off  RndMeth=Floor
  Constant : Constant  Value=struct_EAC_SENS  OutDataTypeStr=Bus: EAC_SENS
  Constant1 : Constant  Value=0
  Enumerated Constant : simulink/Sources/Enumerated Constant  OutDataTypeStr=Enum: SENS_STATUS  Value=SENS_STATUS.OK  SampleTime=inf
  Switch : Switch  Criteria=u2 > Threshold  SaturateOnIntegerOverflow=off  InputSameDT=off
  Terminator : Terminator
  Transfer Fcn2 : TransferFcn  Numerator=[4]  Denominator=[1 2 4]
  EAC_SENS : Outport  OutDataTypeStr=Bus: EAC_SENS  PortDimensions=1
  wires:
  Constant1/1 -> Switch/3
  Switch/1 -> Transfer Fcn2/1
  Cast To Single1/1 -> Bus Assignment2/2
  Cast To Single/1 -> Switch/2, Switch/1
  Bus Selector1/1 -> Bus Assignment2/4  "<s_U_V_EACDCLink_Get>"
  Enumerated Constant/1 -> Bus Assignment2/3
  Transfer Fcn2/1 -> Cast To Single1/1  "s_omega_rpm_EAC_Get"
  EAC_ACT/1 -> Bus Selector/1
  Constant/1 -> Bus Assignment2/1
  Bus Assignment2/1 -> EAC_SENS/1
  Bus Selector/1 -> Cast To Single/1  "<s_omega_rpm_EAC_Set>"
  Bus Selector/2 -> Terminator/1  "<s_Mmax_percent_EAC_Set>"
  s_U_V_EACDCLink_Get/1 -> Bus Selector1/1

== system h2f_175_S2_sil_plant_model/Subsystem4/HVRelays ==
  ElectricalAct : Inport  OutDataTypeStr=Bus: ElectricalAct
  Bus Assignment : BusAssignment  AssignedSignals=s_U_V_EACDCLink_Get
  Bus Selector : BusSelector  OutputSignals=b_HVRelays.s_pos_enum_HVPrePR_Set,b_HVRelays.s_pos_enum_HVPR_Set
  Cast To Single : DataTypeConversion  OutDataTypeStr=single  SaturateOnIntegerOverflow=off  RndMeth=Floor
  Constant : Constant  Value=clean_data_EAC_SENS  OutDataTypeStr=Bus: EAC_SENS
  Constant1 : Constant  Value=0
  Constant2 : Constant  Value=450
  Enumerated Constant : simulink/Sources/Enumerated Constant  OutDataTypeStr=Enum: RELAY_STATE  Value=RELAY_STATE.Connected  SampleTime=inf
  Equal : RelationalOperator  Operator===  OutDataTypeStr=boolean  RndMeth=Simplest  InputSameDT=off
  Equal1 : RelationalOperator  Operator===  OutDataTypeStr=boolean  RndMeth=Simplest  InputSameDT=off
  OR : Logic  Operator=OR  IconShape=distinctive  AllPortsSameDT=off  OutDataTypeStr=boolean
  Switch : Switch  Criteria=u2 > Threshold  SaturateOnIntegerOverflow=off  InputSameDT=off
  b_EAC_SENS : Outport  OutDataTypeStr=Bus: EAC_SENS
  wires:
  Bus Assignment/1 -> b_EAC_SENS/1
  Constant/1 -> Bus Assignment/1
  ElectricalAct/1 -> Bus Selector/1
  Bus Selector/1 -> Equal/2  "<s_pos_enum_HVPrePR_Set>"
  Constant1/1 -> Switch/3
  Constant2/1 -> Switch/1
  Switch/1 -> Cast To Single/1
  Bus Selector/2 -> Equal1/2  "<s_pos_enum_HVPR_Set>"
  Enumerated Constant/1 -> Equal1/1, Equal/1
  Equal/1 -> OR/1
  OR/1 -> Switch/2
  Equal1/1 -> OR/2
  Cast To Single/1 -> Bus Assignment/2

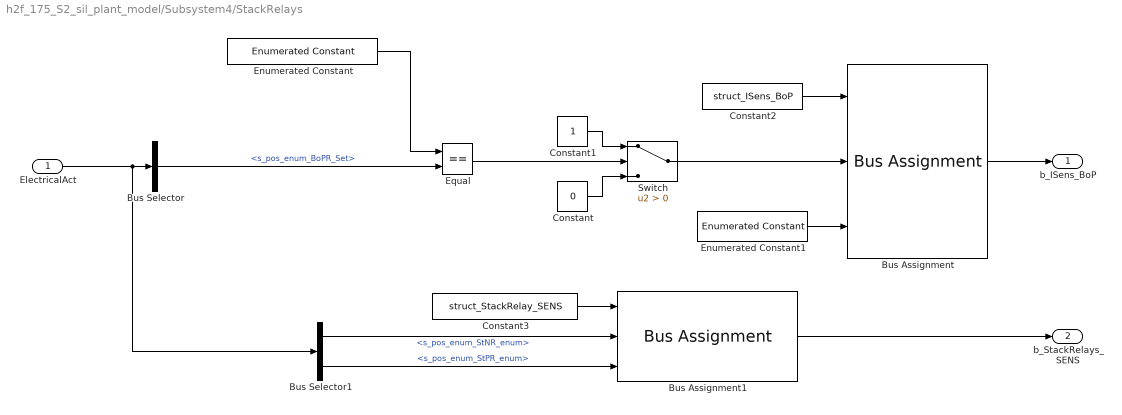
== system h2f_175_S2_sil_plant_model/Subsystem4/StackRelays ==
  ElectricalAct : Inport  OutDataTypeStr=Bus: ElectricalAct
  Bus Assignment : BusAssignment  AssignedSignals=s_I_A_BOP_Get,s_st_enum_BoP_Get
  Bus Assignment1 : BusAssignment  AssignedSignals=s_pos_enum_StNR_Get,s_pos_enum_StPR_Get
  Bus Selector : BusSelector  OutputSignals=b_BoPRelays.s_pos_enum_BoPR_Set
  Bus Selector1 : BusSelector  OutputSignals=b_StackRelays.s_pos_enum_StNR_enum,b_StackRelays.s_pos_enum_StPR_enum
  Constant : Constant  Value=0  OutDataTypeStr=single
  Constant1 : Constant  OutDataTypeStr=single
  Constant2 : Constant  Value=struct_ISens_BoP  OutDataTypeStr=Bus: ISens_BoP
  Constant3 : Constant  Value=struct_StackRelay_SENS  OutDataTypeStr=Bus: StackRelay_SENS
  Enumerated Constant : simulink/Sources/Enumerated Constant  OutDataTypeStr=Enum: RELAY_STATE  Value=RELAY_STATE.Connected  SampleTime=inf
  Enumerated Constant1 : simulink/Sources/Enumerated Constant  OutDataTypeStr=Enum: SENS_STATUS  Value=SENS_STATUS.OK  SampleTime=inf
  Equal : RelationalOperator  Operator===  OutDataTypeStr=boolean  RndMeth=Simplest  InputSameDT=off
  Switch : Switch  Criteria=u2 > Threshold  SaturateOnIntegerOverflow=off  InputSameDT=off
  b_ISens_BoP : Outport  OutDataTypeStr=Bus: ISens_BoP
  b_StackRelays_SENS : Outport  Port=2  OutDataTypeStr=Bus: StackRelay_SENS
  wires:
  Bus Selector/1 -> Equal/2  "<s_pos_enum_BoPR_Set>"
  Enumerated Constant/1 -> Equal/1
  Equal/1 -> Switch/2
  Constant/1 -> Switch/3
  Constant1/1 -> Switch/1
  Constant2/1 -> Bus Assignment/1
  Switch/1 -> Bus Assignment/2
  Bus Assignment/1 -> b_ISens_BoP/1
  Enumerated Constant1/1 -> Bus Assignment/3
  Bus Assignment1/1 -> b_StackRelays_SENS/1
  Bus Selector1/2 -> Bus Assignment1/3  "<s_pos_enum_StPR_enum>"
  Bus Selector1/1 -> Bus Assignment1/2  "<s_pos_enum_StNR_enum>"
  Constant3/1 -> Bus Assignment1/1
  ElectricalAct/1 -> Bus Selector/1, Bus Selector1/1

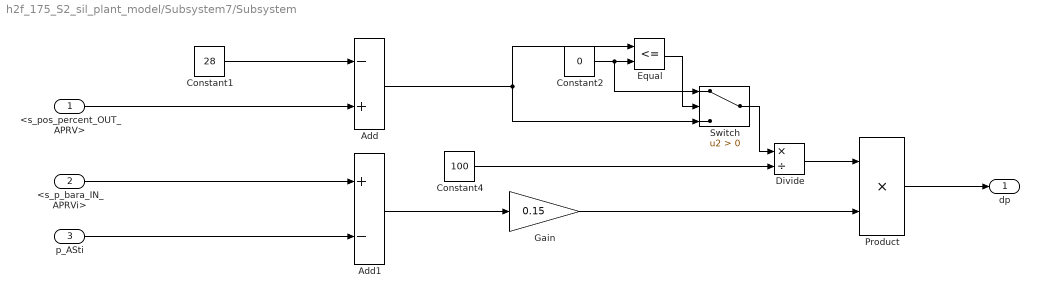
== system h2f_175_S2_sil_plant_model/Subsystem7/Subsystem ==
  <s_pos_percent_OUT_APRV> : Inport
  <s_p_bara_IN_APRVi> : Inport  Port=2
  p_ASti : Inport  Port=3
  Add : Sum  Inputs=-+
  Add1 : Sum  Inputs=+-
  Constant1 : Constant  Value=28  OutDataTypeStr=single
  Constant2 : Constant  Value=0  OutDataTypeStr=single
  Constant4 : Constant  Value=100  OutDataTypeStr=single
  Divide : Product  Inputs=*/
  Equal : RelationalOperator  Operator=<=  OutDataTypeStr=boolean  RndMeth=Simplest  InputSameDT=off
  Gain : Gain  Gain=0.15
  Product : Product
  Switch : Switch  Criteria=u2 > Threshold  SaturateOnIntegerOverflow=off  InputSameDT=off
  dp : Outport
  wires:
  Gain/1 -> Product/2
  Divide/1 -> Product/1
  Add1/1 -> Gain/1
  p_ASti/1 -> Add1/2
  Product/1 -> dp/1
  Constant4/1 -> Divide/2
  <s_p_bara_IN_APRVi>/1 -> Add1/1
  <s_pos_percent_OUT_APRV>/1 -> Add/2
  Add/1 -> Equal/1, Switch/3
  Constant1/1 -> Add/1
  Constant2/1 -> Switch/1, Equal/2
  Equal/1 -> Switch/2
  Switch/1 -> Divide/1

== system h2f_175_S2_sil_plant_model/Subsystem7/h2_consumption ==
  p_ASti : Inport
  Gain : Gain  Gain=-0.0001
  dp : Outport
  wires:
  p_ASti/1 -> Gain/1
  Gain/1 -> dp/1

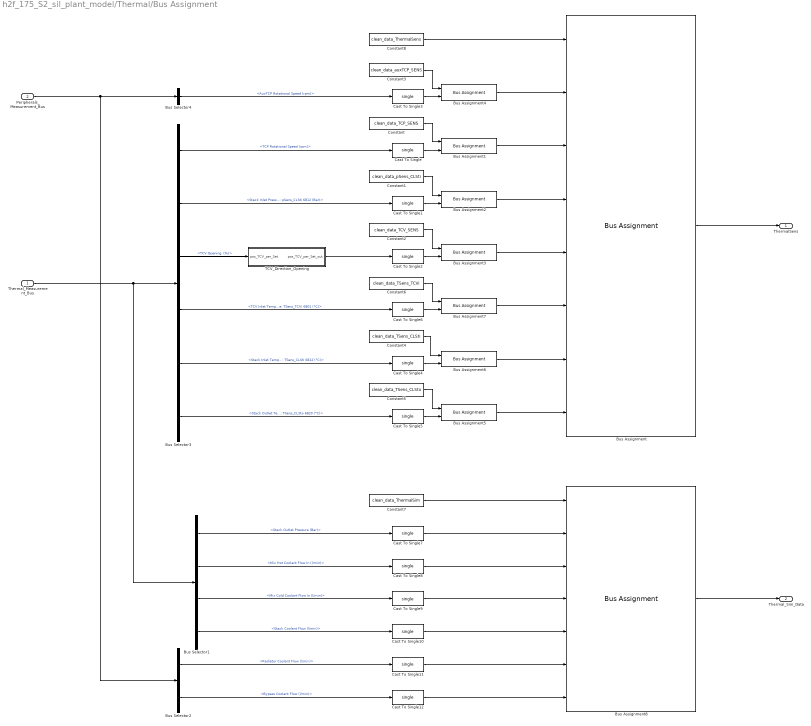
== system h2f_175_S2_sil_plant_model/Thermal/Bus Assignment ==
  Thermal_Measurement_Bus : Inport
  Peripherals_Measurement_Bus : Inport  Port=2
  Bus Assignment : BusAssignment  AssignedSignals=b_auxTCP_SENS,b_TCP_SENS,b_pSens_CLSti,b_TCV_SENS,b_TSens_TCVi,b_TSens_CLSti,b_TSens_CLSto
  Bus Assignment1 : BusAssignment  AssignedSignals=s_omega_rpm_TCP_Get
  Bus Assignment2 : BusAssignment  AssignedSignals=s_p_bara_CLSti_Get
  Bus Assignment3 : BusAssignment  AssignedSignals=s_pos_per_TCV_Get
  Bus Assignment4 : BusAssignment  AssignedSignals=s_omega_rpm_auxTCP_Get
  Bus Assignment5 : BusAssignment  AssignedSignals=s_T_degC_CLSto_Get
  Bus Assignment6 : BusAssignment  AssignedSignals=s_T_degC_CLSti_Get
  Bus Assignment7 : BusAssignment  AssignedSignals=s_T_degC_TCVi_Get
  Bus Assignment8 : BusAssignment  AssignedSignals=s_p_bara_CLSto_Sim,s_VDot_lpm_MixHot_Sim,s_VDot_lpm_MixCold_Sim,s_VDot_lpm_STCL_Sim,s_VDot_lpm_Rad_Sim,s_VDot_lpm_ByP_Sim
  Bus Selector1 : BusSelector  OutputSignals=Stack Outlet Pressure (Bar),Mix Hot Coolant Flow In (l/min),Mix Cold Coolant Flow In (l/min),Stack Coolant Flow (l/min)
  Bus Selector2 : BusSelector  OutputSignals=Radiator Coolant Flow (l/min),Bypass Coolant Flow (l/min)
  Bus Selector3 : BusSelector  OutputSignals="TCP Rotational Speed (rpm),Stack Inlet Pressure: pSens_CLSti 6812 (Bar),TCV Opening  (%),TCV Inlet Temperature: TSens_TCVi 6801 (°C),Stack Inlet Temperature: TSens_CLSti 6812 (°C),Stack Outlet Temperature: TSens_CLSto 6820 (°C)"
  Bus Selector4 : BusSelector  OutputSignals=AuxTCP Rotational Speed (rpm)
  Cast To Single{,1..12} (13 alike) : DataTypeConversion  OutDataTypeStr=single  SaturateOnIntegerOverflow=off  RndMeth=Floor
  Constant : Constant  Value=clean_data_TCP_SENS  OutDataTypeStr=Bus: TCP_SENS
  Constant1 : Constant  Value=clean_data_pSens_CLSti  OutDataTypeStr=Bus: pSens_CLSti
  Constant2 : Constant  Value=clean_data_TCV_SENS  OutDataTypeStr=Bus: TCV_SENS
  Constant3 : Constant  Value=clean_data_auxTCP_SENS  OutDataTypeStr=Bus: auxTCP_SENS
  Constant4 : Constant  Value=clean_data_TSens_CLSti  OutDataTypeStr=Bus: TSens_CLSti
  Constant5 : Constant  Value=clean_data_TSens_CLSto  OutDataTypeStr=Bus: TSens_CLSto
  Constant6 : Constant  Value=clean_data_TSens_TCVi  OutDataTypeStr=Bus: TSens_TCVi
  Constant7 : Constant  Value=clean_data_ThermalSim  OutDataTypeStr=Bus: ThermalSim
  Constant8 : Constant  Value=clean_data_ThermalSens  OutDataTypeStr=Bus: ThermalSens
  TCV_Direction_Opening : Subsystem  Variant=on  VariantActivationTime=startup
  ThermalSens : Outport
  Thermal_Sim_Data : Outport  Port=2  OutDataTypeStr=Bus: ThermalSim
  wires:
  Bus Selector3/2 -> Cast To Single1/1  "<Stack Inlet Pressure: pSens_CLSti 6812 (Bar)>"
  Constant2/1 -> Bus Assignment3/1
  Constant5/1 -> Bus Assignment5/1
  Constant6/1 -> Bus Assignment7/1
  Bus Selector3/3 -> TCV_Direction_Opening/1(pos_TCV_per_Set)  "<TCV Opening  (%)>"
  Cast To Single6/1 -> Bus Assignment7/2
  Cast To Single2/1 -> Bus Assignment3/2
  Cast To Single4/1 -> Bus Assignment6/2
  Bus Assignment5/1 -> Bus Assignment/8
  Constant4/1 -> Bus Assignment6/1
  Constant3/1 -> Bus Assignment4/1
  Constant/1 -> Bus Assignment1/1
  Cast To Single5/1 -> Bus Assignment5/2
  Constant8/1 -> Bus Assignment/1
  Bus Selector3/6 -> Cast To Single5/1  "<Stack Outlet Temperature: TSens_CLSto 6820 (°C)>"
  Thermal_Measurement_Bus/1 -> Bus Selector1/1, Bus Selector3/1
  Bus Assignment2/1 -> Bus Assignment/4
  Bus Selector4/1 -> Cast To Single3/1  "<AuxTCP Rotational Speed (rpm)>"
  Peripherals_Measurement_Bus/1 -> Bus Selector2/1, Bus Selector4/1
  Bus Selector3/4 -> Cast To Single6/1  "<TCV Inlet Temperature: TSens_TCVi 6801 (°C)>"
  Bus Assignment7/1 -> Bus Assignment/6
  Cast To Single/1 -> Bus Assignment1/2
  Bus Selector3/1 -> Cast To Single/1  "<TCP Rotational Speed (rpm)>"
  Cast To Single3/1 -> Bus Assignment4/2
  Constant1/1 -> Bus Assignment2/1
  Cast To Single1/1 -> Bus Assignment2/2
  Bus Assignment/1 -> ThermalSens/1
  Bus Assignment6/1 -> Bus Assignment/7
  Bus Assignment1/1 -> Bus Assignment/3
  Bus Assignment3/1 -> Bus Assignment/5
  Bus Selector3/5 -> Cast To Single4/1  "<Stack Inlet Temperature: TSens_CLSti 6812 (°C)>"
  Bus Assignment4/1 -> Bus Assignment/2
  TCV_Direction_Opening/1(pos_TCV_per_Set_out) -> Cast To Single2/1
  Constant7/1 -> Bus Assignment8/1
  Bus Assignment8/1 -> Thermal_Sim_Data/1
  Bus Selector1/1 -> Cast To Single7/1  "<Stack Outlet Pressure (Bar)>"
  Bus Selector1/2 -> Cast To Single8/1  "<Mix Hot Coolant Flow In (l/min)>"
  Bus Selector1/3 -> Cast To Single9/1  "<Mix Cold Coolant Flow In (l/min)>"
  Bus Selector1/4 -> Cast To Single10/1  "<Stack Coolant Flow (l/min)>"
  Bus Selector2/1 -> Cast To Single11/1  "<Radiator Coolant Flow (l/min)>"
  Bus Selector2/2 -> Cast To Single12/1  "<Bypass Coolant Flow (l/min)>"
  Cast To Single7/1 -> Bus Assignment8/2
  Cast To Single8/1 -> Bus Assignment8/3
  Cast To Single9/1 -> Bus Assignment8/4
  Cast To Single10/1 -> Bus Assignment8/5
  Cast To Single11/1 -> Bus Assignment8/6
  Cast To Single12/1 -> Bus Assignment8/7

== system h2f_175_S2_sil_plant_model/Thermal/TCV_Direction_Opening ==
  pos_TCV_per_Set : Inport
  Open_Leads_To_Cooling : Subsystem  TreatAsAtomicUnit=on  VariantControl=variantConfig.TCVDirection == VARIANT_TCVDirection.OPEN_IS_COOLING
  Open_Leads_To_Heating : Subsystem  TreatAsAtomicUnit=on  VariantControl=variantConfig.TCVDirection == VARIANT_TCVDirection.OPEN_IS_HEATING
  pos_TCV_per_Set_out : Outport

== system h2f_175_S2_sil_plant_model/Thermal/Thermal Subsystem Plant Model ==
  TCV Opening Command (%) : Inport
  TCP Rotational Speed Command (rpm) : Inport  Port=2
  Thermal_Model_Stage_2 : Subsystem  VariantControl=THERMALMODEL_VARIANT_STAGE_TWO  ReferencedSubsystem=thermal_model_stage_2
      settings: PortSchema="{\"entries\":[{\"content\":{\"sides\":[{\"content\":{\"connectorIds\":[\"In1\",\"In2\"]},\"type\":\"ConnectorPlacement.EquallySpacedRectSide\",\"uuid\":\"beafa6ad-25d9-43ec-83ed-6cc27c4ae524\"},{\"content\":{\"connectorIds\":[\"RConn1\",\"RConn2\",\"Out1\"],\"side\":\"RIGHT\"},\"type\":\"ConnectorPlacement.EquallySpacedRectSide\",\"uuid\":\"0e4b084f-16c4-4479-9add-ada13fc3130c\"},{\"content\":{\"connectorIds\":[\"LConn2\",\"LConn1\"],\"side\":\"TOP\"},\"type\":\"ConnectorPlacement.EquallySpacedRectSide\",\"uuid\":\"1a5fc455-48ce-4ccf-a3dc-1364efaff46d\"}]},\"type\":\"ConnectorPlacement.EquallySpacedConnector\",\"uuid\":\"dcdc6280-b7d6-42a7-acf0-0a1a3b6a3e13\"}],\"packageUris\":[\"http://schema.mathworks.com/mf0/Connector/R2020b\"],\"version\":\"1.0\"}"
  Thermal_Model_Stage_2mod : Subsystem  VariantControl=THERMALMODEL_VARIANT_STAGE_TWO_MOD  ReferencedSubsystem=thermal_model_stage_2_mod
      settings: PortSchema="{\"entries\":[{\"content\":{\"sides\":[{\"content\":{\"connectorIds\":[\"In1\",\"In2\"]},\"type\":\"ConnectorPlacement.EquallySpacedRectSide\",\"uuid\":\"beafa6ad-25d9-43ec-83ed-6cc27c4ae524\"},{\"content\":{\"connectorIds\":[\"RConn1\",\"RConn2\",\"Out1\"],\"side\":\"RIGHT\"},\"type\":\"ConnectorPlacement.EquallySpacedRectSide\",\"uuid\":\"0e4b084f-16c4-4479-9add-ada13fc3130c\"},{\"content\":{\"connectorIds\":[\"LConn2\",\"LConn1\"],\"side\":\"TOP\"},\"type\":\"ConnectorPlacement.EquallySpacedRectSide\",\"uuid\":\"1a5fc455-48ce-4ccf-a3dc-1364efaff46d\"}]},\"type\":\"ConnectorPlacement.EquallySpacedConnector\",\"uuid\":\"dcdc6280-b7d6-42a7-acf0-0a1a3b6a3e13\"}],\"packageUris\":[\"http://schema.mathworks.com/mf0/Connector/R2020b\"],\"version\":\"1.0\"}"
  Thermal_Model_Stage_3 : Subsystem  VariantControl=THERMALMODEL_VARIANT_STAGE_THREE  ReferencedSubsystem=thermal_model_stage_3
      settings: PortSchema="{\"entries\":[{\"content\":{\"sides\":[{\"content\":{\"connectorIds\":[\"In1\",\"In2\"]},\"type\":\"ConnectorPlacement.EquallySpacedRectSide\",\"uuid\":\"beafa6ad-25d9-43ec-83ed-6cc27c4ae524\"},{\"content\":{\"connectorIds\":[\"RConn1\",\"RConn2\",\"Out1\"],\"side\":\"RIGHT\"},\"type\":\"ConnectorPlacement.EquallySpacedRectSide\",\"uuid\":\"0e4b084f-16c4-4479-9add-ada13fc3130c\"},{\"content\":{\"connectorIds\":[\"LConn2\",\"LConn1\"],\"side\":\"TOP\"},\"type\":\"ConnectorPlacement.EquallySpacedRectSide\",\"uuid\":\"1a5fc455-48ce-4ccf-a3dc-1364efaff46d\"}]},\"type\":\"ConnectorPlacement.EquallySpacedConnector\",\"uuid\":\"dcdc6280-b7d6-42a7-acf0-0a1a3b6a3e13\"}],\"packageUris\":[\"http://schema.mathworks.com/mf0/Connector/R2020b\"],\"version\":\"1.0\"}"
  Coolant_from_Stack : PMIOPort  Side=Left
  Coolant_to_Stack : PMIOPort  Port=2  Side=Left
  Coolant_to_Peripherals : PMIOPort  Port=3  Side=Right
  Coolant_from_Peripherals : PMIOPort  Port=4  Side=Right
  Thermal_Measurement_Bus : Outport
